simulink model "iap_device_application_demo"  (Simulink 7.3)
settings: Solver=FixedStepDiscrete  SolverMode=SingleTasking  StartTime=0.0  StopTime=10.0  RelTol=1e-3
PreLoadFcn:
  | waijung.modelPreload; % Required for working with Waijung Blockset. Do not remove.
undefined symbols (not defined in the file): HSEOSC, LQFP176, STM32F417IG
libraries: simulink x10, stm32f4_canbus_lib x4, stm32f4_flash_lib x2, stm32f4_io_lib x2, stm32f4_reset_lib x1, stm32f4_device_config_lib x1
CloseFcn:
  | waijung.modelClose; % Required for working with Waijung Blockset. Do not remove.
settings Model: Creator=Krisada  LastModifiedBy=Krisada
settings OptimizationCC: OptimizeModelRefInitCode=on  LifeSpan=1
settings HardwareCC: ProdEndianess=LittleEndian  ProdHWDeviceType=ARM Compatible->Cortex - M4  TargetEndianess=LittleEndian  TargetHWDeviceType=ARM Compatible->Cortex - M4
settings RTWCC: SystemTargetFile=stm32f4.tlc  GenerateMakefile=off  TemplateMakefile=ert_default_tmf  Description=STM32F4 Target  ProcessScript=stm32f4_make_rtw_hook
settings CodeAppCC: IgnoreCustomStorageClasses=off
settings STFCustomTargetCC: ModelReferenceCompliant=off  CombineOutputUpdateFcns=on  ERTCustomFileBanners=on  SupportContinuousTime=off  SupportNonInlinedSFcns=off  SystemTargetFile=stm32f4.tlc
settings ERTTargetCC: MultiwordLength=2048  ModelReferenceCompliant=off  ParMdlRefBuildCompliant=off  CompOptLevelCompliant=off  ERTFirstTimeCompliant=off  ModelStepFunctionPrototypeControlCompliant=off  CPPClassGenCompliant=off  ExtModeMexFile=noextcomm  InlinedParameterPlacement=NonHierarchical  ERTSrcFileBannerTemplate=stm32f4_code_template.cgt  ERTHdrFileBannerTemplate=stm32f4_code_template.cgt  ERTDataSrcFileTemplate=stm32f4_code_template.cgt  ERTDataHdrFileTemplate=stm32f4_code_template.cgt  ERTCustomFileTemplate=stm32f4_file_process.tlc

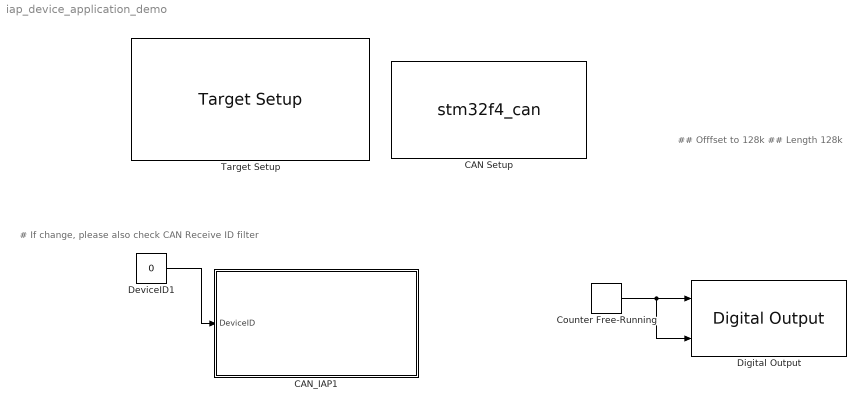
== system iap_device_application_demo ==
  note: ## Offfset to 128k
      | ## Length 128k
  note: # If change,
      | please also check CAN Receive ID filter
  CAN Setup : S-Function  FunctionName=stm32f4_can  Parameters=conf,canmodule,0,inputarray,outputarray,'','',confstr,sampletime,sampletimestr,blockid  EnableBusSupport=off  mask(stm32f4_can){conf=Setup, canmodule=1, advance=on, bitrate_select=125000, sjw=1tq, bs1=14tq, bs2=6tq, timingconf=Prescaler, brp=16, bitrate=125000, tq=3.8095e-007, remaptxpin=B9, remaprxpin=B8, sampletime=inf, sampletimestr=0.001, blockid=CANSetup, inputarray=[], inputlabelarray={}, outputarray=[], outputlabelarray={}, compat=0, confstr=["125000","16","B","9","B","8","1tq","14tq","6tq","ENABLE"], presc=16, txportstr=B, txpinstr=9, rxportstr=B, rxpinstr=8, lastmodule=1}
      mask prompts: conf "Configuration"; canmodule "CAN Module"; advance "Advance configuration"; bitrate_select "Baud rate (bps)"; sjw "Resync Jump Width (SJW)"; bs1 "Bit segment 1 (BS1) + PROP_SEG"; bs2 "Bit segment 2 (BS2)"; timingconf "Adjust"; brp "Baud rate prescaler (BRP)"; bitrate "Baud rate (bps)"; tq "Time Quantum (Second), tq"; remaptxpin "CAN Tx pin"; remaprxpin "CAN Rx pin"; sampletime "Sample time (sec)"; sampletimestr "Compiled sample time (sec) in string"; inputarray "Input port"; inputlabelarray "Input port label"; outputarray "Output port"; outputlabelarray "Output port label"; compat "Compatibility (Reserved for future use)"; confstr "Configuration String"; presc "Prescale"; txportstr "Tx port string"; txpinstr "Tx pin string"; rxportstr "Rx port string"; rxpinstr "Rx pin string"; lastmodule "Last module selected"
      mask help: This block setups CAN Module.
      mask init:
      | stm32f4_can_callback('init');
      mask Help: web(fullfile(waijungdocroot,'stm32f4_can_setup.htm'), '-browser')
      mask StyleString: popup(Setup),popup(1|2),checkbox,popup(125000|250000|500000|1000000),popup(1tq|2tq|3tq|4tq),popup(1tq|2tq|3tq|4tq|5tq|6tq|7tq|8tq|9tq|10tq|11tq|12tq|13tq|14tq|15tq|16tq),popup(1tq|2tq|3tq|4tq|5tq|6tq|7tq|8tq),popup(Prescaler|Baudrate),edit,edit,edit,popup(Not used|A12|B9|D1|H13),popup(Not used|A11|B8|D0|I9),edit,edit,edit,edit,edit,edit,edit,edit,edit,edit,edit,edit,edit,edit,edit
      mask CallbackString: |stm32f4_can_callback('canmodule');|stm32f4_can_callback('advance');|stm32f4_can_callback('bitrate_select');||stm32f4_can_callback('timingconf');|stm32f4_can_callback('timingconf');|stm32f4_can_callback('timingconf');|stm32f4_can_callback('timingconf');|stm32f4_can_callback('timingconf');||stm32f4_can_callback('remaptxpin');|stm32f4_can_callback('remaprxpin');|stm32f4_can_callback('sampletime');|stm32f4_can_callback('sampletimestr');|stm32f4_can_callback('blockid');||||||||||||
      mask Display: text(0.5, 0.5, 'CAN1_Setup\nSpeed (bps): 125000\nTx/Rx pin: B9/B8','ver','middle','hor','center');
  CAN_IAP1 : Subsystem  TreatAsAtomicUnit=on
  Counter Free-Running : simulink/Sources/Counter Free-Running  SystemSampleTime=-1  NumBits=16  tsamp=0.1
  DeviceID1 : Constant  Value=0  OutDataTypeMode=uint32  OutDataType=fixdt(1, 16)  OutScaling=2^0  OutDataTypeStr=uint32  SampleTime=0.001
  Digital Output : stm32f4_io_lib/Digital Output  use_bitband=on  port=D  speed=100  porttype=Push Pull  porttypestr=PP  use_pin0=off  use_pin1=off  use_pin2=off  use_pin3=off  use_pin4=off  use_pin5=off  use_pin6=off  use_pin7=off  use_pin8=off  use_pin9=off  use_pin10=off  use_pin11=off  use_pin12=on  use_pin13=on  use_pin14=off  use_pin15=off  pinstr=GPIO_Pin_12 | GPIO_Pin_13  usedpinarray="[0  0  0  0  0  0  0  0  0  0  0  0  1  1  0  0]"  bitbandingstr=|  sampletime=-1  sampletimestr=0.1  blockid=DigitalOutput  enablecustomportlabel=off  globalinit=off  cinputportlabel=In1, In2  coutputportlabel=0
      | #define DigitalOutput_D12 Peripheral_BB(GPIOD->ODR, 12)  /* Output pin */
      | #define DigitalOutput_D13 Peripheral_BB(GPIOD->ODR, 13)  /* Output pin */
  Target Setup : stm32f4_device_config_lib/Target Setup  Priority=100  compiler=GNU ARM  previous_compiler=GNU ARM  mcu=STM32F417IG (LQFP176)  mcustr=STM32F417IG  clockconfig=HSEOSC-8MHz  system_stm32f4xx_c_path=F:\trunk\targets\stm32f4_target\stm32f4\utils\system_stm32f4xx_default\STM32F40_41xxx\hseosc8mhz  showmemoryconfiguration=off  stacksize=0x2000  heapsize=0x2000  enableautocompiledownload=on  fullchiperase=off  programmerinterface=None  editctrlstr=on  compilercontrolstr=$(patsubst %, -I%, .) -mcpu=cortex-m4 -mthumb -mthumb-interwork -mfloat-abi=hard -mfpu=fpv4-sp-d16 -ffast-math -Wall -Wextra -Ofast  assemblercontrolstr=$(patsubst %, -I%, .) -mcpu=cortex-m4 -mthumb -mthumb-interwork -mfloat-abi=hard -mfpu=fpv4-sp-d16 -ffast-math -Wall -Wextra -Ofast -Wa,-amhls=$(<:.s=.lst) -D__STACK_SIZE=$(STACK_SIZE) -D__HEAP_SIZE=$(HEAP_SIZE)  linkercontrolstr=-T$(LD_SCRIPT) -g -Wl,-Map=$(MAP),--cref,--no-warn-mismatch -mcpu=cortex-m4 -mthumb -mthumb-interwork -mfloat-abi=hard -mfpu=fpv4-sp-d16 -specs=nosys.specs  runafterdownload=on  execprofile=None  profileruart=3  profilerbaud=500000  profilertxpin=D8  profilerinitstr=0.001,168000000,168000,500000,0  manualsetsampletime=off  sampletime=0.001  blockid=TargetSetup  systickreloadvalue=168000  hseval=8000000  lastprofileruart=3  hclk=168000000  flashorigin=0x8000000  flashlength=1024k  ramorigin=0x20000000  ramlength=128k  useextram=off
  wires:
  Counter Free-Running/1 -> Digital Output/1, Digital Output/2
  DeviceID1/1 -> CAN_IAP1/1(DeviceID)

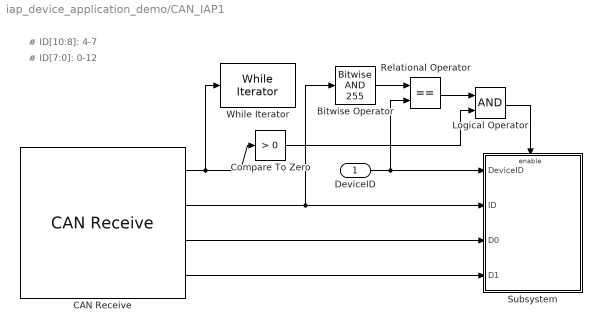
== system iap_device_application_demo/CAN_IAP1 ==
  note: # ID[7:0]: 0-12
  note: # ID[10:8]: 4-7
  DeviceID : Inport  OutDataType=fixdt(1, 16)  OutScaling=2^0
  Bitwise Operator : simulink/Logic and Bit Operations/Bitwise Operator  logicop=AND  UseBitMask=on  BitMask=255  BitMaskRealWorld=Stored Integer
  CAN Receive : stm32f4_canbus_lib/CAN Receive  conf=Rx  canmodule=1  idtype=Standard  filtertype=Mask  id=hex2dec('400')  idmask=hex2dec('4F0')  enableisr=off  usedlc=off  datatype=uint32  data0type=uint32  data1type=uint32  data2type=Not used  data3type=Not used  data4type=Not used  data5type=Not used  data6type=Not used  data7type=Not used  buffersize=32  sampletime=-1  sampletimestr=-1  blockid=CAN_IAP1CANReceive  inputarray=[]  inputlabelarray={}  outputarray=[ 5, 7, 7, 7]  outputlabelarray={ 'Msg Pending','ID', 'D0 (uint32)', 'D1 (uint32)' }  compat=0  confstr="[\"Standard\",\"Mask\",\"1024\",\"1264\",\"off\",\"uint32\",\"uint32\",\"Not used\",\"Not used\",\"Not used\",\"Not used\",\"Not used\",\"Not used\",\"32\",\"8000\",\"0\",\"9E00\",\"4\"]"
  Compare To Zero : simulink/Logic and Bit Operations/Compare To Zero  SystemSampleTime=-1  relop=>  LogicOutDataTypeMode=uint8  ZeroCross=off
  Logical Operator : Logic  AllPortsSameDT=off  OutDataTypeMode=boolean  LogicDataType=fixdt(0, 8)  OutDataTypeStr=boolean
  Relational Operator : RelationalOperator  Operator===  LogicOutDataTypeMode=boolean  LogicDataType=fixdt(0, 8)  OutDataTypeStr=boolean
  Subsystem : Subsystem
  While Iterator : WhileIterator  WhileBlockType=do-while
  wires:
  CAN Receive/1 -> Compare To Zero/1, While Iterator/1
  CAN Receive/4 -> Subsystem/4(D1)
  CAN Receive/2 -> Subsystem/2(ID), Bitwise Operator/1
  CAN Receive/3 -> Subsystem/3(D0)
  Relational Operator/1 -> Logical Operator/1
  Compare To Zero/1 -> Logical Operator/2
  Logical Operator/1 -> Subsystem/Enable
  Bitwise Operator/1 -> Relational Operator/1
  DeviceID/1 -> Subsystem/1(DeviceID), Relational Operator/2

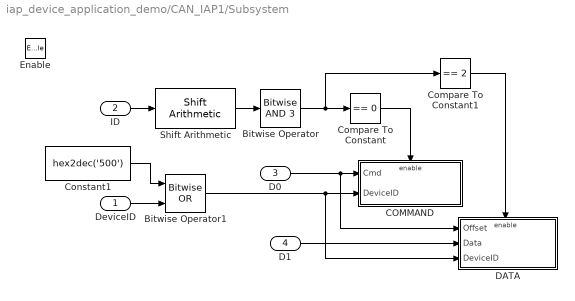
== system iap_device_application_demo/CAN_IAP1/Subsystem ==
  DeviceID : Inport
  ID : Inport  Port=2
  D0 : Inport  Port=3
  D1 : Inport  Port=4
  Enable : EnablePort
  Bitwise Operator : simulink/Logic and Bit Operations/Bitwise Operator  logicop=AND  UseBitMask=on  BitMask=3  BitMaskRealWorld=Stored Integer
  Bitwise Operator1 : simulink/Logic and Bit Operations/Bitwise Operator  logicop=OR  UseBitMask=off  NumInputPorts=2  BitMask=bin2dec('11011001')  BitMaskRealWorld=Stored Integer
  COMMAND : Subsystem  TreatAsAtomicUnit=on
  Compare To Constant : simulink/Logic and Bit Operations/Compare To Constant  SystemSampleTime=-1  relop===  const=0  LogicOutDataTypeMode=uint8  ZeroCross=off
  Compare To Constant1 : simulink/Logic and Bit Operations/Compare To Constant  SystemSampleTime=-1  relop===  const=2  LogicOutDataTypeMode=uint8  ZeroCross=off
  Constant1 : Constant  Value=hex2dec('500')  OutDataTypeMode=uint32  OutDataType=fixdt(1, 16)  OutScaling=2^0  OutDataTypeStr=uint32
  DATA : Subsystem  TreatAsAtomicUnit=on
  Shift Arithmetic : simulink/Logic and Bit Operations/Shift Arithmetic  SystemSampleTime=-1  nBitShiftRight=8  nBinPtShiftRight=0
  wires:
  Shift Arithmetic/1 -> Bitwise Operator/1
  Bitwise Operator/1 -> Compare To Constant1/1, Compare To Constant/1
  Compare To Constant/1 -> COMMAND/Enable
  D0/1 -> COMMAND/1(Cmd), DATA/1(Offset)
  Compare To Constant1/1 -> DATA/Enable
  ID/1 -> Shift Arithmetic/1
  D1/1 -> DATA/2(Data)
  Constant1/1 -> Bitwise Operator1/1
  DeviceID/1 -> Bitwise Operator1/2
  Bitwise Operator1/1 -> COMMAND/2(DeviceID), DATA/3(DeviceID)

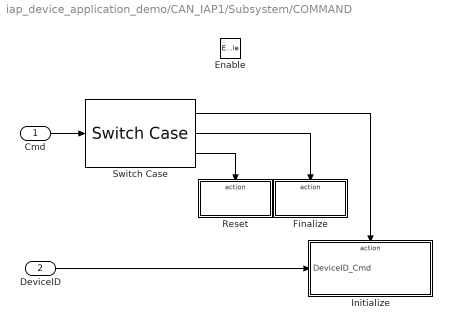
== system iap_device_application_demo/CAN_IAP1/Subsystem/COMMAND ==
  Cmd : Inport  OutDataType=fixdt(1, 16)  OutScaling=2^0
  DeviceID : Inport  Port=2  OutDataType=fixdt(1, 16)  OutScaling=2^0
  Enable : EnablePort
  Finalize : Subsystem  TreatAsAtomicUnit=on
  Initialize : Subsystem  TreatAsAtomicUnit=on
  Reset : Subsystem  TreatAsAtomicUnit=on
  Switch Case : SwitchCase  CaseConditions={0,1,2}  CaseShowDefault=off
  wires:
  Cmd/1 -> Switch Case/1
  Switch Case/1 -> Initialize/Action
  Switch Case/2 -> Finalize/Action
  Switch Case/3 -> Reset/Action
  DeviceID/1 -> Initialize/1(DeviceID_Cmd)

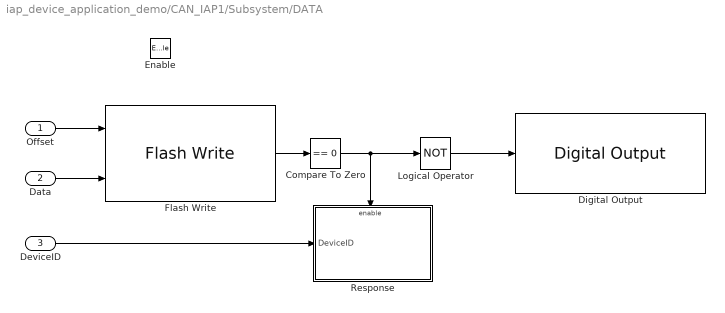
== system iap_device_application_demo/CAN_IAP1/Subsystem/DATA ==
  Offset : Inport  OutDataType=fixdt(1, 16)  OutScaling=2^0
  Data : Inport  Port=2  OutDataType=fixdt(1, 16)  OutScaling=2^0
  DeviceID : Inport  Port=3  OutDataType=fixdt(1, 16)  OutScaling=2^0
  Enable : EnablePort
  Compare To Zero : simulink/Logic and Bit Operations/Compare To Zero  SystemSampleTime=-1  relop===  LogicOutDataTypeMode=uint8  ZeroCross=off
  Digital Output : stm32f4_io_lib/Digital Output  use_bitband=on  port=D  speed=100  porttype=Push Pull  porttypestr=PP  use_pin0=off  use_pin1=off  use_pin2=off  use_pin3=off  use_pin4=off  use_pin5=off  use_pin6=off  use_pin7=off  use_pin8=off  use_pin9=off  use_pin10=off  use_pin11=off  use_pin12=off  use_pin13=off  use_pin14=on  use_pin15=off  pinstr=GPIO_Pin_14  usedpinarray="[0  0  0  0  0  0  0  0  0  0  0  0  0  0  1  0]"  bitbandingstr="#define CAN_IAP1SubsystemDATADigitalOutput_D14 Peripheral_BB(GPIOD->ODR, 14)  /* Output pin */"  sampletime=-1  sampletimestr=-1  blockid=CAN_IAP1SubsystemDATADigitalOutput  enablecustomportlabel=off  globalinit=off  cinputportlabel=In1, In2  coutputportlabel=0
  Flash Write : stm32f4_flash_lib/Flash Write  conf=Program  transfer=Blocking  flashsector=Sector 6: 0x08040000 - 0x0805FFFF  datatype=uint32  datacount=1  enablestatus=on  sampletime=-1  sampletimestr=-1  blockid=CAN_IAP1SubsystemDATAFlashWrite  inputarray=[-1,7]  inputlabelarray={'Offset ', 'Data (uint32)'}  outputarray=[3]  outputlabelarray={'Status'}  compat=0  confstr="[\"Blocking\",\"uint32\",\"on\",\"20000\",\"08040000\",\"6\"]"
  Logical Operator : Logic  Operator=NOT  AllPortsSameDT=off  OutDataTypeMode=boolean  LogicDataType=fixdt(0, 8)  OutDataTypeStr=boolean
  Response : Subsystem
  wires:
  Offset/1 -> Flash Write/1
  Data/1 -> Flash Write/2
  Compare To Zero/1 -> Response/Enable, Logical Operator/1
  Flash Write/1 -> Compare To Zero/1
  DeviceID/1 -> Response/1(DeviceID)
  Logical Operator/1 -> Digital Output/1

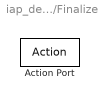
== system iap_device_application_demo/CAN_IAP1/Subsystem/COMMAND/Finalize ==
  Action Port : ActionPort  ActionType=case

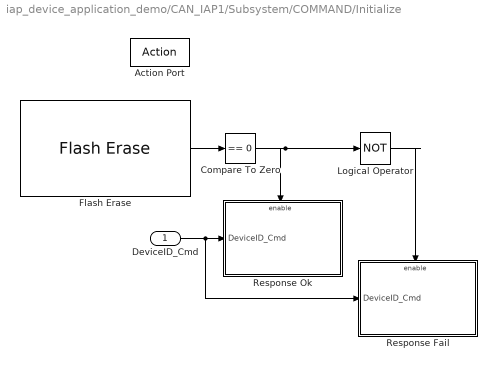
== system iap_device_application_demo/CAN_IAP1/Subsystem/COMMAND/Initialize ==
  DeviceID_Cmd : Inport  OutDataType=fixdt(1, 16)  OutScaling=2^0
  Action Port : ActionPort  ActionType=case
  Compare To Zero : simulink/Logic and Bit Operations/Compare To Zero  SystemSampleTime=-1  relop===  LogicOutDataTypeMode=uint8  ZeroCross=off
  Flash Erase : stm32f4_flash_lib/Flash Erase  conf=Erase  transfer=Blocking  flashsector=Sector 6: 0x08040000 - 0x0805FFFF  datatype=uint32  datacount=1  enablestatus=on  sampletime=-1  sampletimestr=-1  blockid=CAN_IAP1SubsystemCOMMANDInitializeFlashErase  inputarray=[]  inputlabelarray={}  outputarray=[3]  outputlabelarray={'Status'}  compat=0  confstr="[\"Blocking\",\"on\",\"08040000\",\"6\"]"
  Logical Operator : Logic  Operator=NOT  AllPortsSameDT=off  OutDataTypeMode=boolean  LogicDataType=fixdt(0, 8)  OutDataTypeStr=boolean
  Response Fail : Subsystem
  Response Ok : Subsystem
  wires:
  Flash Erase/1 -> Compare To Zero/1
  Compare To Zero/1 -> Response Ok/Enable, Logical Operator/1
  Logical Operator/1 -> Response Fail/Enable
  DeviceID_Cmd/1 -> Response Ok/1(DeviceID_Cmd), Response Fail/1(DeviceID_Cmd)

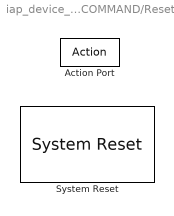
== system iap_device_application_demo/CAN_IAP1/Subsystem/COMMAND/Reset ==
  Action Port : ActionPort  ActionType=case
  System Reset : stm32f4_reset_lib/System Reset  conf=<empty>  sampletime=inf  sampletimestr=-1  blockid=CAN_IAP1SubsystemCOMMANDResetSystemReset  inputarray=[]  inputlabelarray={}  outputarray=[]  outputlabelarray={}  compat=0  confstr="[\"Param1\",\"Param1\"]"

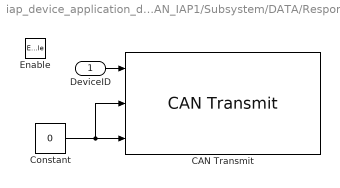
== system iap_device_application_demo/CAN_IAP1/Subsystem/DATA/Response ==
  DeviceID : Inport  OutDataType=fixdt(1, 16)  OutScaling=2^0
  Enable : EnablePort
  CAN Transmit : stm32f4_canbus_lib/CAN Transmit  conf=Tx  canmodule=1  transfer=Blocking  timeout=0.001  idtype=Standard  specificid=off  id=hex2dec('400')  specificdlc=on  dlc=8  enablestatus=off  datatype=uint32  data0type=uint32  data1type=uint32  data2type=Not used  data3type=Not used  data4type=Not used  data5type=Not used  data6type=Not used  data7type=Not used  inputarray=[ -1, 7, 7]  inputlabelarray={ 'ID', 'D0 (uint32)', 'D1 (uint32)' }  outputarray=[]  outputlabelarray={}  sampletime=-1  sampletimestr=-1  blockid=CAN_IAP1SubsystemDATAResponseCANTransmit  compat=0  confstr="[\"Blocking\",\"0.001\",\"Standard\",\"off\",\"1024\",\"on\",\"8\",\"off\",\"uint32\",\"uint32\",\"Not used\",\"Not used\",\"Not used\",\"Not used\",\"Not used\",\"Not used\"]"
  Constant : Constant  Value=0  OutDataTypeMode=uint32  OutDataType=fixdt(1, 16)  OutScaling=2^0  OutDataTypeStr=uint32
  wires:
  DeviceID/1 -> CAN Transmit/1
  Constant/1 -> CAN Transmit/3, CAN Transmit/2

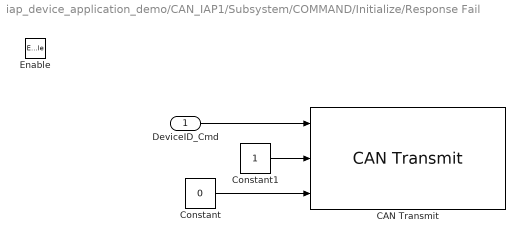
== system iap_device_application_demo/CAN_IAP1/Subsystem/COMMAND/Initialize/Response Fail ==
  DeviceID_Cmd : Inport  OutDataType=fixdt(1, 16)  OutScaling=2^0
  Enable : EnablePort
  CAN Transmit : stm32f4_canbus_lib/CAN Transmit  conf=Tx  canmodule=1  transfer=Blocking  timeout=0.001  idtype=Standard  specificid=off  id=hex2dec('400')  specificdlc=on  dlc=8  enablestatus=off  datatype=uint32  data0type=uint32  data1type=uint32  data2type=Not used  data3type=Not used  data4type=Not used  data5type=Not used  data6type=Not used  data7type=Not used  inputarray=[ -1, 7, 7]  inputlabelarray={ 'ID', 'D0 (uint32)', 'D1 (uint32)' }  outputarray=[]  outputlabelarray={}  sampletime=-1  sampletimestr=-1  blockid=CAN_IAP1SubsystemCOMMANDInitializeResponseFailCANTransmit  compat=0  confstr="[\"Blocking\",\"0.001\",\"Standard\",\"off\",\"1024\",\"on\",\"8\",\"off\",\"uint32\",\"uint32\",\"Not used\",\"Not used\",\"Not used\",\"Not used\",\"Not used\",\"Not used\"]"
  Constant : Constant  Value=0  OutDataTypeMode=uint32  OutDataType=fixdt(1, 16)  OutScaling=2^0  OutDataTypeStr=uint32
  Constant1 : Constant  OutDataTypeMode=uint32  OutDataType=fixdt(1, 16)  OutScaling=2^0  OutDataTypeStr=uint32
  wires:
  Constant/1 -> CAN Transmit/3
  Constant1/1 -> CAN Transmit/2
  DeviceID_Cmd/1 -> CAN Transmit/1

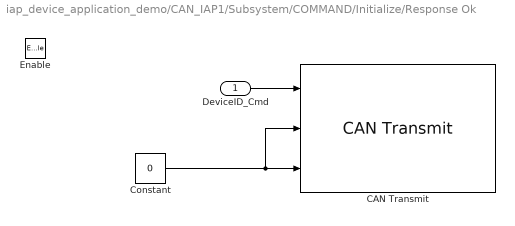
== system iap_device_application_demo/CAN_IAP1/Subsystem/COMMAND/Initialize/Response Ok ==
  DeviceID_Cmd : Inport  OutDataType=fixdt(1, 16)  OutScaling=2^0
  Enable : EnablePort
  CAN Transmit : stm32f4_canbus_lib/CAN Transmit  conf=Tx  canmodule=1  transfer=Blocking  timeout=0.001  idtype=Standard  specificid=off  id=hex2dec('400')  specificdlc=on  dlc=8  enablestatus=off  datatype=uint32  data0type=uint32  data1type=uint32  data2type=Not used  data3type=Not used  data4type=Not used  data5type=Not used  data6type=Not used  data7type=Not used  inputarray=[ -1, 7, 7]  inputlabelarray={ 'ID', 'D0 (uint32)', 'D1 (uint32)' }  outputarray=[]  outputlabelarray={}  sampletime=-1  sampletimestr=-1  blockid=CAN_IAP1SubsystemCOMMANDInitializeResponseOkCANTransmit  compat=0  confstr="[\"Blocking\",\"0.001\",\"Standard\",\"off\",\"1024\",\"on\",\"8\",\"off\",\"uint32\",\"uint32\",\"Not used\",\"Not used\",\"Not used\",\"Not used\",\"Not used\",\"Not used\"]"
  Constant : Constant  Value=0  OutDataTypeMode=uint32  OutDataType=fixdt(1, 16)  OutScaling=2^0  OutDataTypeStr=uint32
  wires:
  Constant/1 -> CAN Transmit/3, CAN Transmit/2
  DeviceID_Cmd/1 -> CAN Transmit/1
